simulink model "Adaptive_control"  (R2023a)
settings: Solver=VariableStepAuto  StartTime=0.0  StopTime=30  RelTol=1e-3
model workspace: external: MAT-File (data not in the file)
undefined symbols (not defined in the file): DiscIntNeverNeededParam, f_s, Kd_ad, Lambda, pi_0
settings Model: Creator=benit  LastModifiedBy=Savio Del Peschio
settings OptimizationCC: ReuseModelBlockBuffer=off

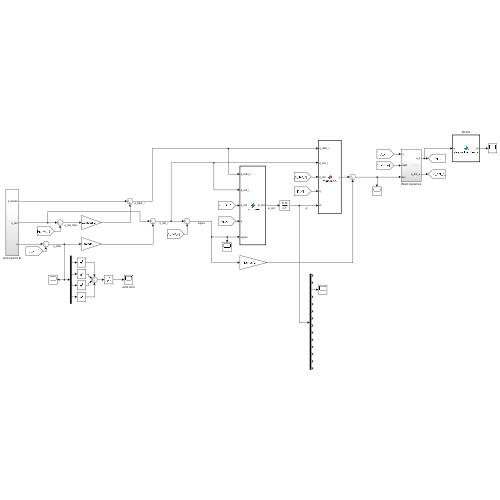
[thumbnail: Simulink's stored preview of the top-level diagram]
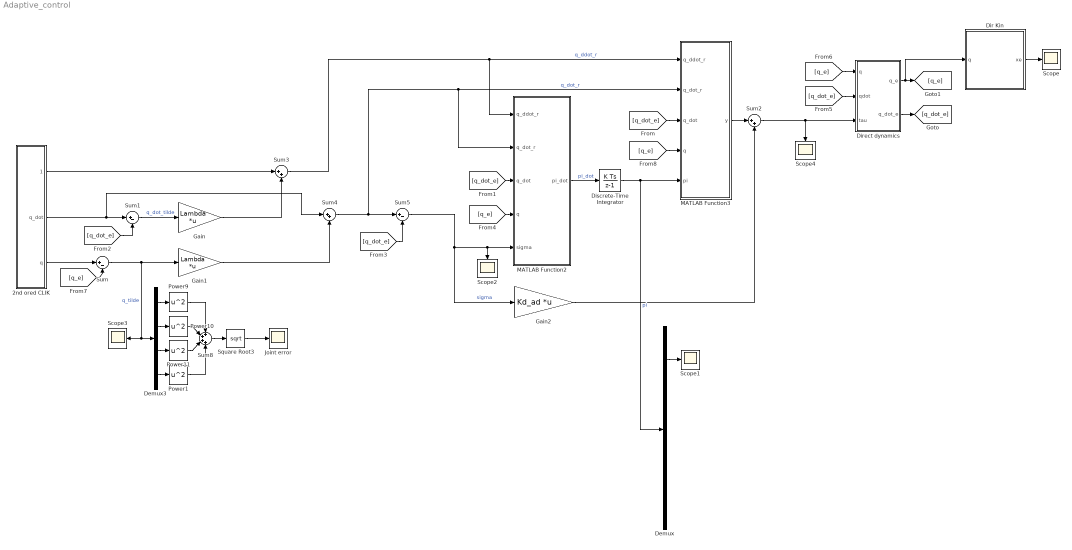
== system Adaptive_control ==
  2nd ored CLIK : Subsystem
  Demux : Demux  Outputs=14
  Demux3 : Demux
  Dir Kin : MATLAB Function  TreatAsAtomicUnit=on
  Direct dynamics : Subsystem
  Discrete-Time Integrator : DiscreteIntegrator  InitialCondition=pi_0  SampleTime=1/f_s  ICPrevOutput=DiscIntNeverNeededParam  ICPrevScaledInput=DiscIntNeverNeededParam
  Gain : Gain  Gain=Lambda  Multiplication=Matrix(K*u)
  Gain1 : Gain  Gain=Lambda  Multiplication=Matrix(K*u)
  Gain2 : Gain  Gain=Kd_ad  Multiplication=Matrix(K*u)
  Joint error : Scope
  MATLAB Function2 : MATLAB Function  TreatAsAtomicUnit=on
  MATLAB Function3 : MATLAB Function  TreatAsAtomicUnit=on
  Power{1,9..11} (4 alike) : Math  Operator=square
  Scope{,1..4} (5 alike) : Scope
  Square Root3 : Sqrt
  Sum : Sum  Inputs=|+-
  Sum1 : Sum  Inputs=|+-
  Sum2 : Sum  Inputs=|++
  Sum3 : Sum  Inputs=|++
  Sum4 : Sum  Inputs=|++
  Sum5 : Sum  Inputs=|+-
  Sum8 : Sum  Inputs=++++
  wires:
  2nd ored CLIK/2(q_dot) -> Sum4/1, Sum1/1
  Sum1/1 -> Gain/1  "q_dot_tilde"
  Sum/1 -> Demux3/1, Scope3/1, Gain1/1  "q_tilde"
  Dir Kin/1(xe) -> Scope/1
  2nd ored CLIK/1(q_dotdot) -> Sum3/1
  Gain/1 -> Sum3/2
  Gain1/1 -> Sum4/2
  Sum4/1 -> MATLAB Function3/2(q_dot_r), MATLAB Function2/2(q_dot_r), Sum5/1  "q_dot_r"
  Sum3/1 -> MATLAB Function3/1(q_ddot_r), MATLAB Function2/1(q_ddot_r)  "q_ddot_r"
  Sum5/1 -> MATLAB Function2/5(sigma), Scope2/1, Gain2/1  "sigma"
  Discrete-Time Integrator/1 -> Demux/1, MATLAB Function3/5(pi)  "pi"
  MATLAB Function3/1(y) -> Sum2/1
  Gain2/1 -> Sum2/2
  MATLAB Function2/1(pi_dot) -> Discrete-Time Integrator/1  "pi_dot"
  Demux3/1 -> Power9/1
  Sum8/1 -> Square Root3/1
  Power10/1 -> Sum8/2
  Power11/1 -> Sum8/3
  Demux3/3 -> Power11/1
  Power9/1 -> Sum8/1
  Demux3/2 -> Power10/1
  Square Root3/1 -> Joint error/1
  Demux3/4 -> Power1/1
  Power1/1 -> Sum8/4
  Direct dynamics/2(q_dot_e) -> [q_dot_e]
  [q_dot_e] -> MATLAB Function3/3(q_dot)
  [q_dot_e] -> MATLAB Function2/3(q_dot)
  [q_dot_e] -> Sum1/2
  [q_dot_e] -> Sum5/2
  Direct dynamics/1(q_e) -> [q_e], Dir Kin/1(q)
  [q_e] -> MATLAB Function2/4(q)
  [q_dot_e] -> Direct dynamics/2(qdot)
  [q_e] -> Direct dynamics/1(q)
  [q_e] -> Sum/2
  [q_e] -> MATLAB Function3/4(q)
  2nd ored CLIK/3(q) -> Sum/1
  Sum2/1 -> Scope4/1, Direct dynamics/3(tau)
  Demux/3 -> Scope1/1

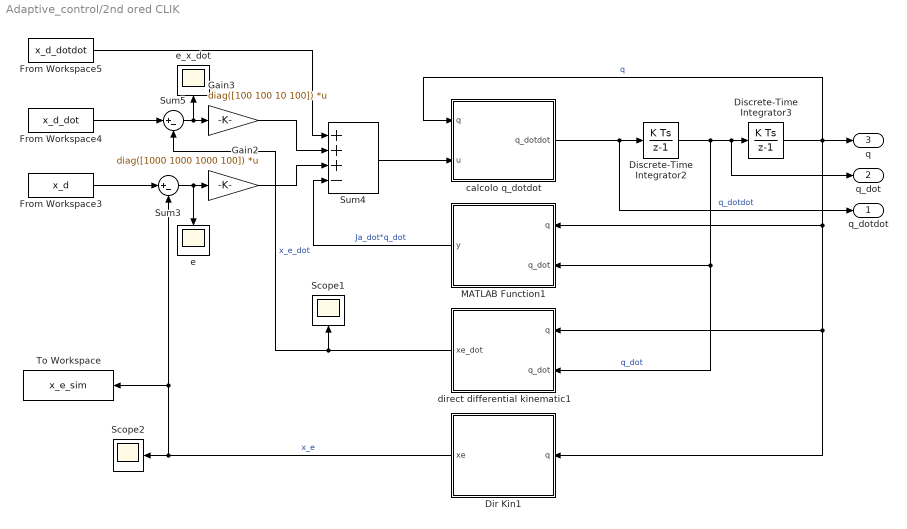
== system Adaptive_control/2nd ored CLIK ==
  Dir Kin1 : MATLAB Function  TreatAsAtomicUnit=on
  Discrete-Time Integrator2 : DiscreteIntegrator  gainval=1  InitialCondition=zeros(4,1)  SampleTime=1/f_s  ICPrevOutput=DiscIntNeverNeededParam  ICPrevScaledInput=DiscIntNeverNeededParam
  Discrete-Time Integrator3 : DiscreteIntegrator  gainval=1  InitialCondition=config_p_init'  SampleTime=1/f_s  ICPrevOutput=DiscIntNeverNeededParam  ICPrevScaledInput=DiscIntNeverNeededParam
  From Workspace3 : FromWorkspace  VariableName=x_d
  From Workspace4 : FromWorkspace  VariableName=x_d_dot
  From Workspace5 : FromWorkspace  VariableName=x_d_dotdot
  Gain2 : Gain  Gain=diag([1000 1000 1000 100])  Multiplication=Matrix(K*u)
  Gain3 : Gain  Gain=diag([100 100 10 100])  Multiplication=Matrix(K*u)
  MATLAB Function1 : MATLAB Function  TreatAsAtomicUnit=on
  Scope1 : Scope
  Scope2 : Scope
  Sum3 : Sum  Inputs=|+-
  Sum4 : Sum  Inputs=+++-
  Sum5 : Sum  Inputs=|+-
  To Workspace : ToWorkspace  VariableName=x_e_sim  SaveFormat=Timeseries  SampleTime=-1
  calcolo q_dotdot : MATLAB Function  TreatAsAtomicUnit=on
  direct differential kinematic1 : MATLAB Function  TreatAsAtomicUnit=on
  e : Scope
  e_x_dot : Scope
  q_dotdot : Outport
  q_dot : Outport  Port=2
  q : Outport  Port=3
  wires:
  Sum4/1 -> calcolo q_dotdot/2(u)
  Discrete-Time Integrator3/1 -> q/1, Dir Kin1/1(q), direct differential kinematic1/1(q), MATLAB Function1/1(q), calcolo q_dotdot/1(q)  "q"
  Dir Kin1/1(xe) -> To Workspace/1, Sum3/2, Scope2/1  "x_e"
  Gain3/1 -> Sum4/2
  From Workspace4/1 -> Sum5/1
  calcolo q_dotdot/1(q_dotdot) -> q_dotdot/1, Discrete-Time Integrator2/1  "q_dotdot"
  From Workspace3/1 -> Sum3/1
  MATLAB Function1/1(y) -> Sum4/4  "Ja_dot*q_dot"
  Gain2/1 -> Sum4/3
  Sum5/1 -> e_x_dot/1, Gain3/1
  From Workspace5/1 -> Sum4/1
  Discrete-Time Integrator2/1 -> direct differential kinematic1/2(q_dot), MATLAB Function1/2(q_dot), q_dot/1, Discrete-Time Integrator3/1  "q_dot"
  direct differential kinematic1/1(xe_dot) -> Sum5/2, Scope1/1  "x_e_dot"
  Sum3/1 -> e/1, Gain2/1

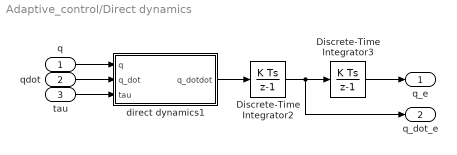
== system Adaptive_control/Direct dynamics ==
  q : Inport
  qdot : Inport  Port=2
  tau : Inport  Port=3
  Discrete-Time Integrator2 : DiscreteIntegrator  InitialCondition=zeros(4,1)  SampleTime=1/f_s  ICPrevOutput=DiscIntNeverNeededParam  ICPrevScaledInput=DiscIntNeverNeededParam
  Discrete-Time Integrator3 : DiscreteIntegrator  InitialCondition=config_p_init'  SampleTime=1/f_s  ICPrevOutput=DiscIntNeverNeededParam  ICPrevScaledInput=DiscIntNeverNeededParam
  direct dynamics1 : MATLAB Function  TreatAsAtomicUnit=on
  q_e : Outport
  q_dot_e : Outport  Port=2
  wires:
  Discrete-Time Integrator2/1 -> q_dot_e/1, Discrete-Time Integrator3/1
  qdot/1 -> direct dynamics1/2(q_dot)
  tau/1 -> direct dynamics1/3(tau)
  Discrete-Time Integrator3/1 -> q_e/1
  direct dynamics1/1(q_dotdot) -> Discrete-Time Integrator2/1
  q/1 -> direct dynamics1/1(q)

== matlab function Adaptive_control/2nd ored CLIK/Dir Kin1 ==
  data: q input; xe output
function xe = cinematica_diretta(q)
    
    xe = [  0.5*cos(q(1))+0.5*cos(q(1)+q(2));
            0.5*sin(q(1))+0.5*sin(q(1)+q(2));
            1/2-q(3)
            q(1)+q(2)-q(4) ];

end

== matlab function Adaptive_control/2nd ored CLIK/MATLAB Function1 ==
  data: q input; q_dot input; y output
function y = Ja_dot(q, q_dot)

    J_min_dot = [-0.5*(q_dot(1)+q_dot(2))*cos(q(1)+q(2))-0.5*q_dot(1)*cos(q(1))              -0.5*(q_dot(1)+q_dot(2))*cos(q(1)+q(2))  0   0
                 -0.5*(q_dot(1)+q_dot(2))*sin(q(1)+q(2))-0.5*q_dot(1)*sin(q(1))              -0.5*(q_dot(1)+q_dot(2))*sin(q(1)+q(2))  0   0
                 0                                                                            0                                       0   0
                 0                                                                            0                                       0   0];
    
     y = J_min_dot*q_dot;
     
end

== matlab function Adaptive_control/2nd ored CLIK/calcolo q_dotdot ==
  data: q input; u input; q_dotdot output
function q_dotdot = fcn(q,u)

    J = [-0.5*sin(q(1))-0.5*sin(q(1)+q(2))   -0.5*sin(q(1)+q(2))    0  0 
          0.5*cos(q(1))+0.5*cos(q(1)+q(2))    0.5*cos(q(1)+q(2))    0  0 
          0                                   0                    -1  0
          1                                   1                     0  -1];
    
    q_dotdot = pinv(J)*u;

end

== matlab function Adaptive_control/2nd ored CLIK/direct differential kinematic1 ==
  data: q input; q_dot input; xe_dot output
function xe_dot = fcn(q,q_dot)

 Ja = [-0.5*sin(q(1))-0.5*sin(q(1)+q(2)) -0.5*sin(q(1)+q(2))    0 0
      0.5*cos(q(1))+0.5*cos(q(1)+q(2))  0.5*cos(q(1)+q(2))     0 0
      0                                0                    -1 0
      1                                1                    0 -1];

xe_dot = Ja*q_dot;

end

== matlab function Adaptive_control/Dir Kin ==
  data: q input; xe output
function xe = cinematica_diretta(q)
    
    xe = [  0.5*cos(q(1))+0.5*cos(q(1)+q(2));
            0.5*sin(q(1))+0.5*sin(q(1)+q(2));
            1/2-q(3)
            q(1)+q(2)-q(4) ];

end

== matlab function Adaptive_control/MATLAB Function2 ==
  data: pi_dot output; q_ddot_r input; q_dot_r input; q_dot input; q input; sigma input
function pi_dot = regressore(q_ddot_r, q_dot_r, q_dot, q, sigma)

    theta_1 = q(1);
    theta_2 = q(2);
    d_3     = q(3);
    theta_4 = q(4);
    theta_dot_1 = q_dot(1);
    theta_dot_2 = q_dot(2);
    d_dot_3     = q_dot(3);
    theta_dot_4 = q_dot(4);
    q_dot_1_r = q_dot_r(1);
    q_dot_2_r = q_dot_r(2);
    q_dot_3_r = q_dot_r(3);
    q_dot_4_r = q_dot_r(4);
    q_ddot_1_r = q_ddot_r(1);
    q_ddot_2_r = q_ddot_r(2);
    q_ddot_3_r = q_ddot_r(3);
    q_ddot_4_r = q_ddot_r(4);
    
    Y = [q_ddot_1_r/16, q_ddot_1_r*(cos(theta_2)/4 + 5/16) + q_ddot_2_r*(cos(theta_2)/8 + 1/16) - q_dot_2_r*((theta_dot_1*sin(theta_2))/8 + (theta_dot_2*sin(theta_2))/8) - (q_dot_1_r*theta_dot_2*sin(theta_2))/8, q_ddot_1_r*(cos(theta_2)/2 + 1/2) + q_ddot_2_r*(cos(theta_2)/4 + 1/4) - q_dot_2_r*((theta_dot_1*sin(theta_2))/4 + (theta_dot_2*sin(theta_2))/4) - (q_dot_1_r*theta_dot_2*sin(theta_2))/4, q_ddot_1_r, q_ddot_1_r + q_ddot_2_r, q_ddot_1_r + q_ddot_2_r - q_ddot_4_r, q_ddot_1_r, q_ddot_1_r + q_ddot_2_r,         q_ddot_1_r + q_ddot_2_r - 50*q_ddot_3_r,        q_ddot_1_r + q_ddot_2_r - 20*q_ddot_4_r, q_dot_1_r,         0,         0,         0;
                     0,                                                                                                q_ddot_2_r/16 + q_ddot_1_r*(cos(theta_2)/8 + 1/16) + (q_dot_1_r*theta_dot_1*sin(theta_2))/8,                                                                                                q_ddot_2_r/4 + q_ddot_1_r*(cos(theta_2)/4 + 1/4) + (q_dot_1_r*theta_dot_1*sin(theta_2))/4,          0, q_ddot_1_r + q_ddot_2_r, q_ddot_1_r + q_ddot_2_r - q_ddot_4_r,          0, q_ddot_1_r + q_ddot_2_r,         q_ddot_1_r + q_ddot_2_r - 50*q_ddot_3_r,        q_ddot_1_r + q_ddot_2_r - 20*q_ddot_4_r,         0, q_dot_2_r,         0,         0;
                     0,                                                                                                                                                                                          0,                                                                                                                                                                     q_ddot_3_r - 981/100,          0,                       0,                                    0,          0,                       0, 2500*q_ddot_3_r - 50*q_ddot_2_r - 50*q_ddot_1_r,                                              0,         0,         0, q_dot_3_r,         0;
                     0,                                                                                                                                                                                          0,                                                                                                                                                                                        0,          0,                       0, q_ddot_4_r - q_ddot_2_r - q_ddot_1_r,          0,                       0,                                               0, 400*q_ddot_4_r - 20*q_ddot_2_r - 20*q_ddot_1_r,         0,         0,         0, q_dot_4_r];
    
    K_pi = diag([1 1 0.001 1 1 1 1 1 1 1 1 1 1 1])*10;
    
    pi_dot = inv(K_pi)*(Y')*sigma;

end

== matlab function Adaptive_control/MATLAB Function3 ==
  data: q_ddot_r input; y output; q_dot_r input; q_dot input; q input; pi input
function y = regressore(q_ddot_r, q_dot_r, q_dot, q, pi)

    theta_1 = q(1);
    theta_2 = q(2);
    d_3     = q(3);
    theta_4 = q(4);
    theta_dot_1 = q_dot(1);
    theta_dot_2 = q_dot(2);
    d_dot_3     = q_dot(3);
    theta_dot_4 = q_dot(4);
    q_dot_1_r = q_dot_r(1);
    q_dot_2_r = q_dot_r(2);
    q_dot_3_r = q_dot_r(3);
    q_dot_4_r = q_dot_r(4);
    q_ddot_1_r = q_ddot_r(1);
    q_ddot_2_r = q_ddot_r(2);
    q_ddot_3_r = q_ddot_r(3);
    q_ddot_4_r = q_ddot_r(4);

    Y = [q_ddot_1_r/16, q_ddot_1_r*(cos(theta_2)/4 + 5/16) + q_ddot_2_r*(cos(theta_2)/8 + 1/16) - q_dot_2_r*((theta_dot_1*sin(theta_2))/8 + (theta_dot_2*sin(theta_2))/8) - (q_dot_1_r*theta_dot_2*sin(theta_2))/8, q_ddot_1_r*(cos(theta_2)/2 + 1/2) + q_ddot_2_r*(cos(theta_2)/4 + 1/4) - q_dot_2_r*((theta_dot_1*sin(theta_2))/4 + (theta_dot_2*sin(theta_2))/4) - (q_dot_1_r*theta_dot_2*sin(theta_2))/4, q_ddot_1_r, q_ddot_1_r + q_ddot_2_r, q_ddot_1_r + q_ddot_2_r - q_ddot_4_r, q_ddot_1_r, q_ddot_1_r + q_ddot_2_r,         q_ddot_1_r + q_ddot_2_r - 50*q_ddot_3_r,        q_ddot_1_r + q_ddot_2_r - 20*q_ddot_4_r, q_dot_1_r,         0,         0,         0;
                     0,                                                                                                q_ddot_2_r/16 + q_ddot_1_r*(cos(theta_2)/8 + 1/16) + (q_dot_1_r*theta_dot_1*sin(theta_2))/8,                                                                                                q_ddot_2_r/4 + q_ddot_1_r*(cos(theta_2)/4 + 1/4) + (q_dot_1_r*theta_dot_1*sin(theta_2))/4,          0, q_ddot_1_r + q_ddot_2_r, q_ddot_1_r + q_ddot_2_r - q_ddot_4_r,          0, q_ddot_1_r + q_ddot_2_r,         q_ddot_1_r + q_ddot_2_r - 50*q_ddot_3_r,        q_ddot_1_r + q_ddot_2_r - 20*q_ddot_4_r,         0, q_dot_2_r,         0,         0;
                     0,                                                                                                                                                                                          0,                                                                                                                                                                     q_ddot_3_r - 981/100,          0,                       0,                                    0,          0,                       0, 2500*q_ddot_3_r - 50*q_ddot_2_r - 50*q_ddot_1_r,                                              0,         0,         0, q_dot_3_r,         0;
                     0,                                                                                                                                                                                          0,                                                                                                                                                                                        0,          0,                       0, q_ddot_4_r - q_ddot_2_r - q_ddot_1_r,          0,                       0,                                               0, 400*q_ddot_4_r - 20*q_ddot_2_r - 20*q_ddot_1_r,         0,         0,         0, q_dot_4_r];
    
    y=Y*pi;

end

== matlab function Adaptive_control/Direct dynamics/direct dynamics1 ==
  data: q input; q_dot input; q_dotdot output; tau input
function q_dotdot = fcn(q, q_dot, tau)
        
    %attriti dei motori
    Fm_1 = 0.00005;
    Fm_2 = 0.00005;
    Fm_3 = 0.01;
    Fm_4 = 0.005;
    
    theta_2 = q(2);
    theta_dot_1 = q_dot(1);
    theta_dot_2 = q_dot(2);
    d_dot_3 = q_dot(3);
    theta_dot_4 = q_dot(4);
    
    B_p = [(25*cos(theta_2))/2 + 12013/500, (25*cos(theta_2))/4 + 1252/125, -1/4, -51/50;
            (25*cos(theta_2))/4 + 1252/125,                       1252/125, -1/4, -51/50;
                                      -1/4,                           -1/4, 55/2,      0;
                                    -51/50,                         -51/50,    0,    7/5];                                                                                                        
       
    C_p = [-(25*theta_dot_2*sin(theta_2))/4, - (25*theta_dot_1*sin(theta_2))/4 - (25*theta_dot_2*sin(theta_2))/4, 0, 0;
            (25*theta_dot_1*sin(theta_2))/4,                                                                   0, 0, 0;
                                          0,                                                                   0, 0, 0;
                                          0,                                                                   0, 0, 0];
    
    
    F_v = diag([-Fm_1 -Fm_2 -Fm_3 -Fm_4]);
    g = [0, 0, - 9.81*(5+10), 0]';
    tau_primo = C_p*q_dot+F_v*q_dot+g;
    
    q_dotdot = inv(B_p)*(tau-tau_primo); 

end
